simulink model "Delay_test_send"  (R2020a)
settings: Solver=FixedStepAuto  StartTime=0.0  StopTime=inf  RelTol=1e-3  EnableMultiTasking=on
libraries: svdutilitieslib x1, arduinolib x1
settings Model: SILPILModeSetting=veronly  ExtModeTrigDuration=2  Creator=imkis  LastModifiedBy=imkis
settings OptimizationCC: DefaultUnderspecifiedDataType=single  EnhancedBackFolding=on  PassReuseOutputArgsAs=Individual arguments  ZeroExternalMemoryAtStartup=off  ZeroInternalMemoryAtStartup=off  MaxStackSize=64  OptimizeBlockOrder=speed  DifferentSizesBufferReuse=on  EfficientTunableParamExpr=on
settings DebuggingCC: ParameterPrecisionLossMsg=none  ParameterTunabilityLossMsg=error
settings HardwareCC: ProdBitPerInt=16  ProdBitPerPointer=16  ProdBitPerSizeT=16  ProdBitPerPtrDiffT=16  ProdLargestAtomicFloat=None  ProdWordSize=8  ProdHWDeviceType=Atmel->AVR
settings SFSimCC: MATLABDynamicMemAlloc=off
settings RTWCC: SystemTargetFile=ert.tlc  HardwareBoard=Arduino Mega 2560  TLCOptions=-aInlineSetEventsForThisBaseRateFcn=TLC_FALSE -aSuppressMultiTaskScheduler=TLC_FALSE -aRateBasedStepFcn=1  TemplateMakefile=ert_default_tmf  Toolchain=Arduino AVR  BuildConfiguration=Faster Runs
settings CodeAppCC: ForceParamTrailComments=on  IgnoreCustomStorageClasses=off  OperatorAnnotations=on  SimulinkDataObjDesc=on  SFDataObjDesc=on  InsertBlockDesc=on
settings ERTTargetCC: TargetLangStandard=C99 (ISO)  SupportContinuousTime=on  SupportVariableSizeSignals=on  ExtModeStaticAllocSize=2048
settings ConfigComp: PLC_TargetIDE=codesys23

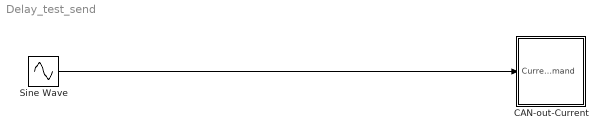
== system Delay_test_send ==
  CAN-out-Current : Subsystem
  Sine Wave : Sin  SineType=Sample based  Amplitude=5000  Samples=0.03/0.001  SampleTime=0.001
  wires:
  Sine Wave/1 -> CAN-out-Current/1("Current Command ")

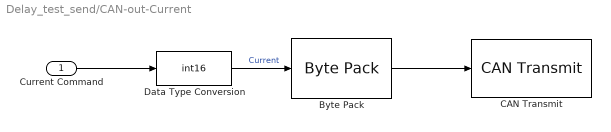
== system Delay_test_send/CAN-out-Current ==
  "Current Command " : Inport
  Byte Pack : svdutilitieslib/Byte Pack  maskPackedDataType=uint8  datatypes={'int16'}  byteAlign=2  blockPlatform=arduinoert
      settings: SourceProductBaseCode=ARDUINO,ML_ARDUINO,ECCORTEXA,ECCORTEXR,SC_BEAGLEBONE_BLUE,EC_FREEDOM_BOARD,EC_FRDM_K64F,INTEL_BLOCKSET,MICROBIT,NUCLEO,PX4AUTOPILOTS,RASPPIIO,STMICRODIS,TIC2000,XILINX_BLOCKSET
  CAN Transmit : arduinolib/CAN Transmit  inputDataType=Raw data  BlockingMode_=off  BlockTimeout_=1  outputStatus=off  identifierType=Standard (11-bit identifier)  messageId=hex2dec('201')  msgLength=2  remoteFrame=off
      settings: SourceProductBaseCode=ARDUINO
  Data Type Conversion : DataTypeConversion  OutDataTypeStr=int16
  wires:
  Data Type Conversion/1 -> Byte Pack/1  "Current"
  Byte Pack/1 -> CAN Transmit/1
  "Current Command "/1 -> Data Type Conversion/1
